simulink model "Latest_Greatest_vSandberg"  (R2022b)
settings: Solver=ode4  StartTime=0  StopTime=15  FixedStep=DeltaT  RelTol=1e-6  EnableMultiTasking=on
InitFcn:
  | %run('final_report_initexternal')
  | % Bifocal Relay Mirror Spacecraft (prior to payload installation) Dynamics Simulation          TA Sands
  | clear all;close all;clc;warning off all;
  | 
  | % Simulation run parameters
  | Rate=34.3; Rate=100;  DeltaT=1/Rate;
  | 
  | % Maneuver Parameters
  | roll=0;  pitch=0; yaw=30;   roll=roll*pi/180; pitch=pitch*pi/180; yaw=yaw*pi/180;
  | SlewStart=5; SlewTime=10; SACengage=0;
  | SlewStart=5; SlewTime=5;
  | t0=SlewTime;
  | tf=SlewTime+5;
  | %%
  | 
  | %Constants0
  | Re=6371.2e3;mu=398601.2e9;          %earth radius and universal gravitation constant
  | 
  | % tht=0.5*((sin(pi/SlewTime*(u(4)+2.5)))+1).*[u(1) u(2) u(3)]';
  | % w=(30/77.1239)*0.5*(pi/SlewTime)*((cos(pi/SlewTime*(u(4)+2.5)))+1).*[u(1) u(2) u(3)]'
  | % wdot=-(30/77.1239)*0.5*(pi/SlewTime)^(2)*((sin(pi/SlewTime*(u(4)+2.5)))).*[u(1) u(2) u(3)]'
  | 
  | %compare with differentiating in real time
  | 
  | % A0=[0 0 0];
  | % tht=A0+1/2*(1-cos(pi/SlewTime*(t-SlewStart)))*(A-A0);
  | % w=1/2*(pi/SlewTime)*sin(pi/SlewTime*(t-SlewStart))*(A-A0);
  | % wdot1=1/2*(pi/SlewTime)^2*cos(pi/SlewTime*(t-SlewStart))*(A-A0);
  | 
  | %Spacecraft orbit
  | h=0;                                     %orbit altitude
  | R=Re+h;                             %orbit radius from center of earth
  | we=0.000072921158553;   %earth's angular velocity rad/solar sec(Vallado)
  | wo=sqrt(mu/(Re+h)^3);        %orbit angular velocity
  | incln=36.6001*pi/180;          %Inclination assumed Monterey Latitude
  | epsilon=12*pi/180;  alphao=0;
  | uo=0; nuo=0;                        %Start S/C beneath subsolar point
  | betasun=60; gamma=1.5;
  | a=0.545491852; b=0.314939867;  c=0.704226952;   %Assumed spacecraft rectangular size
  | Area=[b*c a*c a*b];                 %projected area~m^2 in body x,y,z directions
  | density=4.39e-14;
  | kpre=-9.9639/24/3600/180*pi*0;      %nodal precession constant assumed zero here
  | wn=kpre*(Re/(Re+h))^3.5*cos(incln); %nodal precession (zero eccentricity)
  | V=wo*(Re+h);
  | rho=asin(Re/(h+Re));                %earth angular radius
  | Cd=2.5;     psun=4.5E-6;            %Drag coefficient and solar pressure constant~N/m^2
  | Kaero=-0.5*Cd*V^2;   Psolar=2*psun;  %constants for aero and solar torque calculation
  | dL=[0.002 0.002 0.008];             %predicted distance between cp and cg
  | Kme=2.3390e-005;
  | 
  | %Spacecraft Magnetic Properties (assumed)
  | mresid=[0 0 0.01];                  %Spacecraft residual magnetic moment
  | M=mresid;                           %Magnetic unit dipole vector
  | K=7.943e15;
  | 
  | %%
  | % Determining Principal Axes Frame
  | % ACTUAL Spacecraft Inertia conditions
  | Ix=16.67;   Iy=16.67;   Iz=16.67 ;
  | Ixy=0;  Iyz=0;  Ixz=0;
  | ... (+176 lines)
StopFcn:
  | toc
  | %run('final_report_stopexternal')
  | 
  | if flag==0; Hcmg=Hcmg;else;Hcmg=HcmgMP;end;
  | Hxcmg=[];Hycmg=[];Hzcmg=[];CondA=[]; CondA_MP=[];t=[]; SingPt=[];DetA=[];
  | for i=1:max(size(A));  t=[t i*DeltaT];  H=Hcmg(:,:,i); Hx=H(1,:);  Hy=H(2,:);  Hz=H(3,:);
  | detA=det(A(:,1:3,i));Hxcmg=[Hxcmg Hx];  Hycmg=[Hycmg Hy];  Hzcmg=[Hzcmg Hz];
  | CONDA=cond(A(:,:,i));
  | DetA=[DetA detA]; DetA=1./DetA;
  | CondA=[CondA CONDA];end;   %CondA=CondA./max(CondA); DetA=DetA./max(DetA);
  | Hmag=sqrt(Hxcmg.^2+Hycmg.^2+Hzcmg.^2);x=(max(t)-DeltaT);
  | 
  | InvCondA;
  | 
  | if flag==0; MaxInvCond=min(1./CondA(10*Rate+1:end));DELTA=delta;DELTAdot=deltadot;
  | else; MaxInvCond=min(1./CondA_MP(10*Rate+1:end));DELTA=delta_MP;DELTAdot=deltadot_MP;Hcmg=HcmgMP;end;
  | %
  | ERROR=(trajectory*180/pi-Euler);
  | 
  | figure(1); wdotTrajectory=[CMDTrajectory(:,1) CMDTrajectory(:,2) CMDTrajectory(:,3)];  wTrajectory=[CMDTrajectory(:,4) CMDTrajectory(:,5) CMDTrajectory(:,6)]; ThetaTrajectory=180/pi.*[trajectory(:,1) trajectory(:,2) trajectory(:,3)]; set(gca,'fontsize',32, 'fontname','Palatino Linotype');
  | subplot(3,1,1); plot(t,wdotTrajectory, 'linewidth',2); axis tight; grid; ylabel('\omega^d^o^t_C_M_D (deg)','fontsize',32); title('Desired Angle, Rate, Acceleration Trajectories','fontsize',32);   set(gca,'XTick',0:2:15);     set(gca,'XTickLabel',{' ',' ',' ',' ',' ',' ',' ',' ','15'}); set(gca,'fontsize',32, 'fontname','Palatino Linotype');
  | subplot(3,1,2); plot(t,wTrajectory,'linewidth',2); axis tight; grid; ylabel('\omega_C_M_D (deg)','fontsize',32);set(gca,'XTick',0:2:15);     set(gca,'XTickLabel',{' ',' ',' ',' ',' ',' ',' ',' ','15'}); set(gca,'fontsize',32, 'fontname','Palatino Linotype');
  | subplot(3,1,3); plot(t,ThetaTrajectory,'linewidth',2); axis tight; grid; ylabel('\theta_C_M_D (deg)','fontsize',32); xlabel('time (sec)','fontsize',32); set(gca,'fontsize',32, 'fontname','Palatino Linotype');
  | 
  | % figure(2);
  | % subplot(2,1,1);plot(t,Hmag,'LineWidth',3);   ylabel('|H_c_m_g|','Fontsize',16);grid;axis([0,x,0,3]); set(gca,'fontsize',16);set(gca,'XTickLabel',{' ',' ',' ',' ',' ',' ',' ',' ','15'});
  | % subplot(2,1,2);plot(t,InvCondA,'linewidth',3);grid;xlabel('t(sec)','fontsize',14,'fontname','times');ylabel('Cond[A]','fontsize',14,'fontname','times');axis([0,max(t),0,21.82]); set(gca,'fontsize',16);
  | %
  | % DELTA1=DELTA(1,:);DELTA2=DELTA(2,:);DELTA3=DELTA(3,:);DELTA4=DELTA(4,:);
  | % DELTAdot1=DELTAdot(1,:);DELTAdot2=DELTAdot(2,:);DELTAdot3=DELTAdot(3,:);DELTAdot4=DELTAdot(4,:);
  | %
  | % figure(3);subplot(4,1,1);plot(t,DELTA1,'LineWidth',3); title('Gimbal Angles','fontsize',16);ylabel('\theta_1(deg)','Fontsize',14);grid;axis tight; set(gca,'XTickLabel',{' ',' ',' ',' ',' ',' ',' ',' ','15'});set(gca,'fontsize',16);
  | % subplot(4,1,2);plot(t,DELTA2,'LineWidth',3); ylabel('\theta_2(deg)','Fontsize',16);grid;axis tight; set(gca,'XTickLabel',{' ',' ',' ',' ',' ',' ',' ',' ','15'});set(gca,'fontsize',16);
  | % subplot(4,1,3);plot(t,DELTA3,'LineWidth',3); ylabel('\theta_3(deg)','Fontsize',16);grid;axis tight; set(gca,'XTickLabel',{' ',' ',' ',' ',' ',' ',' ',' ','15'});set(gca,'fontsize',16);
  | % subplot(4,1,4);plot(t,InvCondA,'linewidth',3);grid;xlabel('t(sec)','fontsize',14,'fontname','times');ylabel('Cond[A]','fontsize',14,'fontname','times');axis([0,max(t),0,21.82]); set(gca,'fontsize',16);
  | %
  | % figure(4);subplot(4,1,1);plot(t,DELTAdot1,'LineWidth',3);  title('Gimbal Angle RATES','fontsize',16); ylabel('\theta_d_o_t_1(rad/s)','Fontsize',16);grid; axis([0,x,-pi*1.1,pi*1.1]);   set(gca,'XTickLabel',{' ',' ',' ',' ',' ',' ',' ',' ','15'});set(gca,'fontsize',16);
  | % subplot(4,1,2);plot(t,DELTAdot2,'LineWidth',3);   ylabel('\theta_d_o_t_2(rad/s)','Fontsize',16);grid;axis([0,x,-pi*1.1,pi*1.1]);   set(gca,'XTickLabel',{' ',' ',' ',' ',' ',' ',' ',' ','15'});   set(gca,'fontsize',16);
  | % subplot(4,1,3);plot(t,DELTAdot3,'LineWidth',3);   ylabel('\theta_d_o_t_3(rad/s)','Fontsize',16);grid;axis([0,x,-pi*1.1,pi*1.1]); set(gca,'XTickLabel',{' ',' ',' ',' ',' ',' ',' ',' ','15'});set(gca,'fontsize',16);
  | % subplot(4,1,4);plot(t,InvCondA,'linewidth',3);grid;xlabel('t(sec)','fontsize',14,'fontname','times');ylabel('Cond[A]','fontsize',14,'fontname','times');axis([0,max(t),0,21.82]); set(gca,'fontsize',16);
  | %
  | % figure(5);
  | % subplot(4,1,1);plot(t,Hxcmg,'linewidth',3);axis([0,x,-3.25,3.25]);grid;ylabel('h_x/|h|','fontsize',16);title('Normalized Momentum','fontsize',16);set(gca,'XTickLabel',{' ',' ',' ',' ',' ',' ',' ',' ','15'});set(gca,'fontsize',16);
  | % subplot(4,1,2);plot(t,Hycmg,'linewidth',3);axis([0,x,-3.25,3.25]);grid;ylabel('h_y/|h|','fontsize',16);set(gca,'XTickLabel',{' ',' ',' ',' ',' ',' ',' ',' ','15'});set(gca,'fontsize',16);
  | % subplot(4,1,3);plot(t,Hzcmg,'linewidth',3);axis([0,x,-3.25,3.25]);grid;ylabel('h_z/|h|','fontsize',16);  set(gca,'XTickLabel',{' ',' ',' ',' ',' ',' ',' ',' ','15'});set(gca,'fontsize',16);
  | % subplot(4,1,4);plot(t,InvCondA,'linewidth',3);grid;xlabel('t(sec)','fontsize',14,'fontname','times');ylabel('Cond[A]','fontsize',14,'fontname','times');axis([0,max(t),0,21.82]); set(gca,'fontsize',16);
  | %
  | figure(6); EulerX=Euler(:,1);EulerY=Euler(:,2);EulerZ=Euler(:,3);
  | subplot(4,1,1);plot(t,EulerX,'linewidth',3); axis([0,x,min(EulerX),max(EulerX)]);grid;ylabel('\phi(deg)','fontsize',32);title('True Euler Angles','fontsize',14);  set(gca,'XTickLabel',{' ',' ',' ',' ',' ',' ',' ',' ','15'});  set(gca,'fontsize',32, 'fontname','Palatino Linotype');
  | subplot(4,1,2);plot(t,EulerY,'linewidth',3);  axis([0,x,min(EulerY),max(EulerY)]); grid;ylabel('\theta(deg)','fontsize',32);  set(gca,'XTickLabel',{' ',' ',' ',' ',' ',' ',' ',' ','15'}); set(gca,'fontsize',32, 'fontname','Palatino Linotype');
  | subplot(4,1,3);plot(t,EulerZ,'linewidth',3);axis([0,x,min(EulerZ),max(EulerZ)]);grid;  ylabel('\psi(deg)','fontsize',32);  set(gca,'XTickLabel',{' ',' ',' ',' ',' ',' ',' ',' ','15'});  set(gca,'fontsize',32, 'fontname','Palatino Linotype');
  | subplot(4,1,4);plot(t,InvCondA,'linewidth',3);grid;xlabel('t(sec)','fontsize',32,'fontname','times');ylabel('Cond[A]','fontsize',14,'fontname','times');axis([0,max(t),0,21.82]); set(gca,'fontsize',32, 'fontname','Palatino Linotype');
  | 
  | EX=ERROR(:,1);  EY=ERROR(:,2);     EZ=ERROR(:,3);
  | MeanXerror=mean(EX); Xmean=num2str(MeanXerror); xmean=['\mu_\phi=', Xmean];
  | STDx=std(EX);Xsigma=num2str(STDx);SigmaX=['    \sigma_x=' Xsigma];  xlegend=[xmean, SigmaX];
  | MeanYerror=mean(EY); Ymean=num2str(MeanYerror); ymean=['\mu_\theta=', Ymean];
  | STDy=std(EY); Ysigma=num2str(STDy);SigmaY=['    \sigma_y=' Ysigma]; ylegend=[ymean, SigmaY];
  | MeanZerror=mean(EZ); Zmean=num2str(MeanZerror); zmean=['\mu_\psi=', Zmean];
  | STDz=std(EZ);Zsigma=num2str(STDz);SigmaZ=['    \sigma_z=' Zsigma]; zlegend=[zmean, SigmaZ];
  | ... (+113 lines)
undefined symbols (not defined in the file): magnitude, svd
libraries: vrlib x9, dspinverses x8, aerospace x5, matrix_library x4, simulink_need_slupdate x2, dspadpt3 x2
(part 2 of 4)

== system Latest_Greatest_vSandberg/Subsystem2/Subsystem1 ==
  note: DCM
  note: DCM
  note: Density needs to be fixed
  DCM : Inport
  r_body : Inport  Port=2
  Display : Display
  Gain : Gain
  Gravity Gradient1 : Subsystem
  Magnetic Torque : Subsystem
  On/Off : Gain  SaturateOnIntegerOverflow=on  OutDataTypeStr=Inherit: Same as input  ParamDataTypeStr=Inherit: Same as input
  "On/Off " : Gain  SaturateOnIntegerOverflow=on  OutDataTypeStr=Inherit: Same as input  ParamDataTypeStr=Inherit: Same as input
  On/off : Gain  SaturateOnIntegerOverflow=on  OutDataTypeStr=Inherit: Same as input  ParamDataTypeStr=Inherit: Same as input
  On/off1 : Gain  SaturateOnIntegerOverflow=on  OutDataTypeStr=Inherit: Same as input  ParamDataTypeStr=Inherit: Same as input
  Orbit parameters : Subsystem
  Scope : Scope
  TAero & Tsolar : Subsystem
  Magnetic Disturbance : Outport
  Aero & Solar Disturbances : Outport  Port=2
  Gravity Gradient Disturbance : Outport  Port=3
  Aero & Solar Disturbance Forces : Outport  Port=4
  Gravity Gradient Disturbance Force : Outport  Port=5
  wires:
  Gravity Gradient1/2(Fgg) -> Gain/1, Display/1, Scope/1
  On/off1/1 -> Aero & Solar Disturbance Forces/1
  r_body/1 -> Gravity Gradient1/2(r_body)
  Gravity Gradient1/1(Tgg) -> "On/Off "/1
  Gain/1 -> Gravity Gradient Disturbance Force/1
  TAero & Tsolar/2(Faero & Fsolar1) -> On/off1/1
  "On/Off "/1 -> Gravity Gradient Disturbance/1
  On/off/1 -> Aero & Solar Disturbances/1
  On/Off/1 -> Magnetic Disturbance/1
  Magnetic Torque/1(Sb) -> On/Off/1
  Orbit parameters/3(u) -> Magnetic Torque/4(u)
  Orbit parameters/2(incln) -> Magnetic Torque/3(inclination)
  Orbit parameters/1(alpha) -> Magnetic Torque/2(alpha)
  Orbit parameters/4(nu) -> TAero & Tsolar/1(nu)
  TAero & Tsolar/1(Taero & Tsolar) -> On/off/1
  DCM/1 -> Gravity Gradient1/1(DCM), TAero & Tsolar/2(DCM), Magnetic Torque/1(DCM)

== system Latest_Greatest_vSandberg/Subsystem3/Body Dynamics ==
  note: w
  note: N B
  note: Hs
  note: Hsdot
  note: [ ]
  note: Mx
      | My
      | Mz
  note: [ ]
  note: w
      | w
      | w
  note: x
      | y
      | z
  note: Spacecraft Dynamics
  T : Inport
  Cross Product : matrix_library/Cross Product
  H * Iinv : Gain  Gain=Iinv  Multiplication=Matrix(K*u)  SaturateOnIntegerOverflow=on  OutDataTypeStr=Inherit: Same as input  ParamDataTypeStr=Inherit: Same as input
  Hdot * Iinv : Gain  Gain=Iinv  Multiplication=Matrix(K*u)  SaturateOnIntegerOverflow=on  OutDataTypeStr=Inherit: Same as input  ParamDataTypeStr=Inherit: Same as input
  Integrator : Integrator
  Sum1 : Sum  Inputs=|++  InputSameDT=on  SaturateOnIntegerOverflow=on  OutDataTypeStr=Inherit: Same as first input
  To Workspace1 : ToWorkspace  VariableName=w  SampleTime=-1
  To Workspace2 : ToWorkspace  VariableName=wdot  SampleTime=-1
  h*[A] : Gain  Gain=1/h_wheel
  |H| : Fcn  Expr=sqrt(u[1]^2+u[2]^2+u[3]^2)
  |H| Display : Display
  |H| Scope : Scope
  NwB : Outport  VectorParamsAs1DForOutWhenUnconnected=off
  NwBdot : Outport  Port=2  VectorParamsAs1DForOutWhenUnconnected=off
  tag scope: hxw=global
  wires:
  Integrator/1 -> H * Iinv/1, Cross Product/1, |H|/1
  H * Iinv/1 -> Cross Product/2, NwB/1, To Workspace1/1
  Cross Product/1 -> [hxw], Sum1/2
  |H|/1 -> |H| Display/1, h*[A]/1
  Sum1/1 -> Integrator/1, Hdot * Iinv/1
  T/1 -> Sum1/1
  h*[A]/1 -> |H| Scope/1
  Hdot * Iinv/1 -> NwBdot/1, To Workspace2/1

== system Latest_Greatest_vSandberg/Subsystem3/Subsystem1 ==
  note: [ ]
  note: w
      | w
      | w
  note: x
      | y
      | z
  note: w
  note: N B
  note: w
  note: [ ]
  note: w
      | w
      | w
  note: 1
      | 2
      | 3
  note: w
  note: O B
  note: DCM
  note: N O
  note: [ ]
  note: f
      | q
      | y
  note: Spacecraft Kinematics
  wbn : Inport
  -wo : Gain  Gain=-wo  SaturateOnIntegerOverflow=on  OutDataTypeStr=Inherit: Same as input  ParamDataTypeStr=Inherit: Same as input
  -wo1 : Gain  Gain=0  SaturateOnIntegerOverflow=on  OutDataTypeStr=Inherit: Same as input  ParamDataTypeStr=Inherit: Same as input
  Euler Angle : Subsystem
  Quaternion Kinematics : Subsystem
  Select ci2 : Subsystem
  Sum : Sum  Inputs=-+|  InputSameDT=on  SaturateOnIntegerOverflow=on  OutDataTypeStr=Inherit: Same as first input
  To Workspace : ToWorkspace  VariableName=Euler  SampleTime=-1
  rad2deg : Gain  Gain=180/pi  SaturateOnIntegerOverflow=on  OutDataTypeStr=Inherit: Same as input  ParamDataTypeStr=Inherit: Same as input
  DCM : Outport  VectorParamsAs1DForOutWhenUnconnected=off
  Euler(deg) : Outport  Port=2  VectorParamsAs1DForOutWhenUnconnected=off
  Euler(rad) : Outport  Port=3  VectorParamsAs1DForOutWhenUnconnected=off
  wires:
  Sum/1 -> Quaternion Kinematics/1(OwB)
  -wo/1 -> -wo1/1
  Select ci2/1(U(E)) -> -wo/1
  Quaternion Kinematics/1(DCM) -> Euler Angle/1(DCM1), Select ci2/1(U), DCM/1
  -wo1/1 -> Sum/1
  wbn/1 -> Sum/2
  Euler Angle/1(Euler Angles1) -> rad2deg/1, Euler(rad)/1
  rad2deg/1 -> Euler(deg)/1, To Workspace/1

== system Latest_Greatest_vSandberg/Subsystem5/OBSERVERS (MASK THIS SUBSYSTEM AS CLASS DEMO)1 ==
  Full State Feedback : Inport
  Demux : Demux  Outputs=2
  Subsystem : Subsystem
      mask Display: disp('Luenberger & PID Observers')
  Terminator : Terminator
  Estimated full state feedback (Euler-rad) : Outport  VectorParamsAs1DForOutWhenUnconnected=off
  wires:
  Demux/1 -> Subsystem/1(Euler Angle (rad))
  Demux/2 -> Terminator/1
  Subsystem/1(Estimated Full State Feedback) -> Estimated full state feedback (Euler-rad)/1
  Full State Feedback/1 -> Demux/1

== system Latest_Greatest_vSandberg/Subsystem5/Subsystem2 ==
  note: Noisy Sensor
  Full State Feedback : Inport
  Random Number : RandomNumber  Variance=NoiseVariance  SampleTime=0
  Sum1 : Sum  Inputs=|++
  Noisy State Feedback : Outport  VectorParamsAs1DForOutWhenUnconnected=off
  wires:
  Random Number/1 -> Sum1/2
  Sum1/1 -> Noisy State Feedback/1
  Full State Feedback/1 -> Sum1/1

== system Latest_Greatest_vSandberg/Subsystem5/Subsystem4 ==
  Full State Feedback : Inport
  Demux : Demux  Outputs=2
  Filter Error (deg) : Scope
      settings: StopFcn=|
      | %Simulink figure properties
      | shh=get(0,'ShowHiddenHandles');
      | set(0,'ShowHiddenHandles','On')
      | set(gcf,'menubar','figure')
      | set(gcf,'CloseRequestFcn','closereq')
      | set(gcf,'DefaultLineClipping','Off')
      | set(0,'ShowHiddenHandles',shh)
  Filtered Euler Angles (deg) : Scope
      settings: StopFcn=|
      | %Simulink figure properties
      | shh=get(0,'ShowHiddenHandles');
      | set(0,'ShowHiddenHandles','On')
      | set(gcf,'menubar','figure')
      | set(gcf,'CloseRequestFcn','closereq')
      | set(gcf,'DefaultLineClipping','Off')
      | set(0,'ShowHiddenHandles',shh)
  Kalman Filter : dspadpt3/Kalman Filter  num_targets=1  sourceEnable=Always  isReset=on  X=zeros([3, 1])  P=10*eye(3)  A=eye(3)  sourceMeasure=Specify via Dialog  H=eye(3)  Q=0.05*eye(3)  R=eye(3)  isOutputEstMeasure=off  isOutputEstState=on  isOutputEstError=off  isOutputPrdMeasure=off  isOutputPrdState=off  isOutputPrdError=off
  Kalman Filter1 : dspadpt3/Kalman Filter  num_targets=1  sourceEnable=Always  isReset=on  X=zeros([3, 1])  P=10*eye(3)  A=eye(3)  sourceMeasure=Specify via Dialog  H=eye(3)  Q=0.05*eye(3)  R=eye(3)  isOutputEstMeasure=off  isOutputEstState=on  isOutputEstError=off  isOutputPrdMeasure=off  isOutputPrdState=off  isOutputPrdError=off
  Mux : Mux  Inputs=2
  Reshape : Reshape
  Sum3 : Sum  Inputs=|+-
  To Workspace : ToWorkspace  VariableName=FilteredEuler  SampleTime=-1
  To Workspace2 : ToWorkspace  VariableName=KalmanEstimationError  SampleTime=-1
  degrees-to-radians2 : Gain  Gain=180/pi
  Out1 : Outport  VectorParamsAs1DForOutWhenUnconnected=off
  wires:
  [ActualEuler] -> Sum3/1
  Reshape/1 -> Sum3/2
  Sum3/1 -> Filter Error (deg)/1, To Workspace2/1
  degrees-to-radians2/1 -> Reshape/1, To Workspace/1, Filtered Euler Angles (deg)/1
  Kalman Filter/1 -> degrees-to-radians2/1, Mux/1
  Demux/2 -> Kalman Filter1/1
  Full State Feedback/1 -> Demux/1
  Demux/1 -> Kalman Filter/1
  Mux/1 -> Out1/1
  Kalman Filter1/1 -> Mux/2

== system Latest_Greatest_vSandberg/Subsystem5/Subsystem5 ==
  note: See Bong Wie
      | Generalized Second Order Filters
      | 2nd Edition pg 137
  u : Inport
  Demux : Demux  Outputs=6
  Mux : Mux  Inputs=6
  Transfer Fcn{,1..5} (6 alike) : TransferFcn  Numerator="[1/wz^2   2*dampZ/wz  1]"  Denominator="[1/wp^2   2*dampP/wp  1]"
  u(filtered) : Outport  VectorParamsAs1DForOutWhenUnconnected=off
  wires:
  Mux/1 -> u(filtered)/1
  u/1 -> Demux/1
  Transfer Fcn/1 -> Mux/1
  Transfer Fcn1/1 -> Mux/2
  Transfer Fcn2/1 -> Mux/3
  Transfer Fcn3/1 -> Mux/4
  Transfer Fcn4/1 -> Mux/5
  Transfer Fcn5/1 -> Mux/6
  Demux/1 -> Transfer Fcn/1
  Demux/2 -> Transfer Fcn1/1
  Demux/3 -> Transfer Fcn2/1
  Demux/4 -> Transfer Fcn3/1
  Demux/5 -> Transfer Fcn4/1
  Demux/6 -> Transfer Fcn5/1

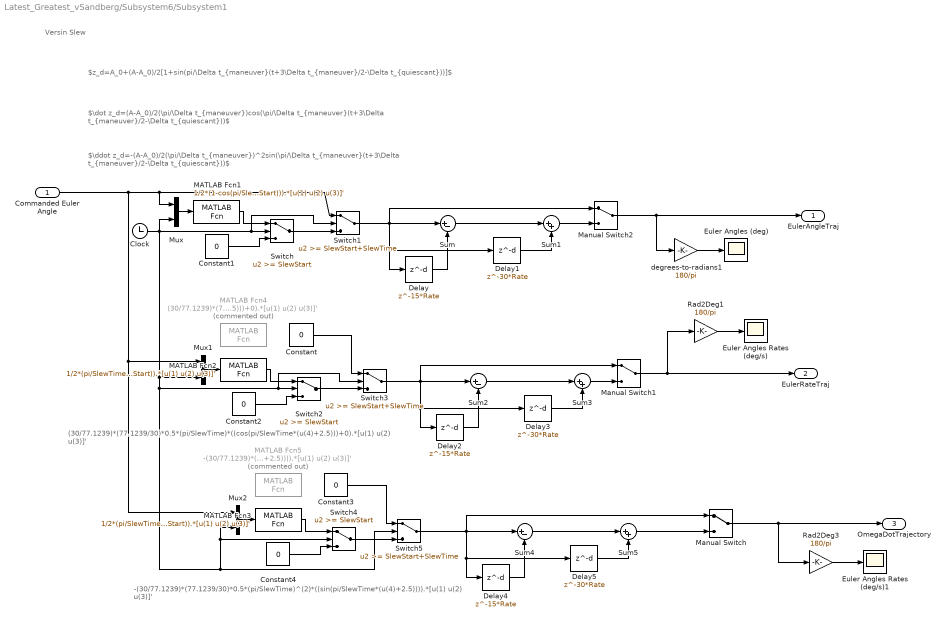
== system Latest_Greatest_vSandberg/Subsystem6/Subsystem1 ==
  note: (30/77.1239)*(77.1239/30)*0.5*(pi/SlewTime)*((cos(pi/SlewTime*(u(4)+2.5)))+0).*[u(1) u(2) u(3)]'
  note: -(30/77.1239)*(77.1239/30)*0.5*(pi/SlewTime)^(2)*((sin(pi/SlewTime*(u(4)+2.5)))).*[u(1) u(2) u(3)]'
  note: Versin Slew
  note: $z_d=A_0+(A-A_0)/2[1+sin(pi/\Delta t_{maneuver}(t+3\Delta t_{maneuver}/2-\Delta t_{quiescant}))]$
  note: $\dot z_d=(A-A_0)/2(\pi/\Delta t_{maneuver})cos(\pi/\Delta t_{maneuver}(t+3\Delta t_{maneuver}/2-\Delta t_{quiescant}))$
  note: $\ddot z_d=-(A-A_0)/2(\pi/\Delta t_{maneuver})^2sin(\pi/\Delta t_{maneuver}(t+3\Delta t_{maneuver}/2-\Delta t_{quiescant}))$
  Commanded Euler Angle : Inport
  Clock : Clock
  Constant{,1..4} (5 alike) : Constant  Value=0
  Delay : Delay  DelayLength=15*Rate
  Delay1 : Delay  DelayLength=30*Rate
  Delay2 : Delay  DelayLength=15*Rate
  Delay3 : Delay  DelayLength=30*Rate
  Delay4 : Delay  DelayLength=15*Rate
  Delay5 : Delay  DelayLength=30*Rate
  Euler Angles (deg) : Scope
      settings: StopFcn=|
      | %Simulink figure properties
      | shh=get(0,'ShowHiddenHandles');
      | set(0,'ShowHiddenHandles','On')
      | set(gcf,'menubar','figure')
      | set(gcf,'CloseRequestFcn','closereq')
      | set(gcf,'DefaultLineClipping','Off')
      | set(0,'ShowHiddenHandles',shh)
  Euler Angles Rates (deg/s) : Scope
      settings: StopFcn=|
      | %Simulink figure properties
      | shh=get(0,'ShowHiddenHandles');
      | set(0,'ShowHiddenHandles','On')
      | set(gcf,'menubar','figure')
      | set(gcf,'CloseRequestFcn','closereq')
      | set(gcf,'DefaultLineClipping','Off')
      | set(0,'ShowHiddenHandles',shh)
  Euler Angles Rates (deg/s)1 : Scope
      settings: StopFcn=|
      | %Simulink figure properties
      | shh=get(0,'ShowHiddenHandles');
      | set(0,'ShowHiddenHandles','On')
      | set(gcf,'menubar','figure')
      | set(gcf,'CloseRequestFcn','closereq')
      | set(gcf,'DefaultLineClipping','Off')
      | set(0,'ShowHiddenHandles',shh)
  MATLAB Fcn1 : MATLABFcn  MATLABFcn=1/2*(1-cos(pi/SlewTime*(u(4)-SlewStart))).*[u(1) u(2) u(3)]'
  MATLAB Fcn2 : MATLABFcn  MATLABFcn=1/2*(pi/SlewTime)*sin(pi/SlewTime*(u(4)-SlewStart)).*[u(1) u(2) u(3)]'
  MATLAB Fcn3 : MATLABFcn  MATLABFcn=1/2*(pi/SlewTime)^2*cos(pi/SlewTime*(u(4)-SlewStart)).*[u(1) u(2) u(3)]'
  MATLAB Fcn4 : MATLABFcn  Commented=on  MATLABFcn=(30/77.1239)*(77.1239/30)*0.5*(pi/SlewTime)*((cos(pi/SlewTime*(u(4)+2.5)))+0).*[u(1) u(2) u(3)]'
  MATLAB Fcn5 : MATLABFcn  Commented=on  MATLABFcn=-(30/77.1239)*(77.1239/30)*0.5*(pi/SlewTime)^(2)*((sin(pi/SlewTime*(u(4)+2.5)))).*[u(1) u(2) u(3)]'
  Manual Switch : ManualSwitch
  Manual Switch1 : ManualSwitch
  Manual Switch2 : ManualSwitch
  Mux : Mux  Inputs=2
  Mux1 : Mux  Inputs=2
  Mux2 : Mux  Inputs=2
  Rad2Deg1 : Gain  Gain=180/pi
  Rad2Deg3 : Gain  Gain=180/pi
  Sum : Sum  Inputs=|+-
  Sum1 : Sum  Inputs=|++
  Sum2 : Sum  Inputs=|+-
  Sum3 : Sum  Inputs=|++
  Sum4 : Sum  Inputs=|+-
  Sum5 : Sum  Inputs=|++
  Switch : Switch  Threshold=SlewStart  SaturateOnIntegerOverflow=off  InputSameDT=off
  Switch1 : Switch  Threshold=SlewStart+SlewTime  SaturateOnIntegerOverflow=off  InputSameDT=off
  Switch2 : Switch  Threshold=SlewStart  SaturateOnIntegerOverflow=off  InputSameDT=off
  Switch3 : Switch  Threshold=SlewStart+SlewTime  SaturateOnIntegerOverflow=off  InputSameDT=off
  Switch4 : Switch  Threshold=SlewStart  SaturateOnIntegerOverflow=off  InputSameDT=off
  Switch5 : Switch  Threshold=SlewStart+SlewTime  SaturateOnIntegerOverflow=off  InputSameDT=off
  degrees-to-radians1 : Gain  Gain=180/pi
  EulerAngleTraj : Outport  VectorParamsAs1DForOutWhenUnconnected=off
  EulerRateTraj : Outport  Port=2  VectorParamsAs1DForOutWhenUnconnected=off
  OmegaDotTrajectory : Outport  Port=3  VectorParamsAs1DForOutWhenUnconnected=off
  wires:
  Mux2/1 -> MATLAB Fcn3/1
  MATLAB Fcn3/1 -> Switch4/1
  Constant4/1 -> Switch4/3
  Switch4/1 -> Switch5/3
  Constant3/1 -> Switch5/1
  Constant/1 -> Switch3/1
  Switch2/1 -> Switch3/3
  Constant2/1 -> Switch2/3
  MATLAB Fcn2/1 -> Switch2/1
  Mux1/1 -> MATLAB Fcn2/1
  Rad2Deg1/1 -> Euler Angles Rates (deg/s)/1
  degrees-to-radians1/1 -> Euler Angles (deg)/1
  Mux/1 -> MATLAB Fcn1/1
  Commanded Euler Angle/1 -> Mux2/1, Mux1/1, Switch1/1, Mux/1
  MATLAB Fcn1/1 -> Switch/1
  Clock/1 -> Switch5/2, Switch4/2, Mux2/2, Switch2/2, Switch3/2, Mux1/2, Mux/2, Switch1/2, Switch/2
  Constant1/1 -> Switch/3
  Switch/1 -> Switch1/3
  Switch1/1 -> Manual Switch2/1, Sum/1, Delay/1, Delay1/1
  Rad2Deg3/1 -> Euler Angles Rates (deg/s)1/1
  Delay/1 -> Sum/2
  Sum/1 -> Sum1/1
  Delay1/1 -> Sum1/2
  Delay2/1 -> Sum2/2
  Delay3/1 -> Sum3/2
  Switch3/1 -> Manual Switch1/1, Sum2/1, Delay2/1, Delay3/1
  Sum2/1 -> Sum3/1
  Delay4/1 -> Sum4/2
  Delay5/1 -> Sum5/2
  Switch5/1 -> Sum4/1, Manual Switch/1, Delay4/1, Delay5/1
  Sum4/1 -> Sum5/1
  Manual Switch/1 -> Rad2Deg3/1, OmegaDotTrajectory/1
  Sum5/1 -> Manual Switch/2
  Manual Switch1/1 -> EulerRateTraj/1, Rad2Deg1/1
  Sum3/1 -> Manual Switch1/2
  Sum1/1 -> Manual Switch2/2
  Manual Switch2/1 -> EulerAngleTraj/1, degrees-to-radians1/1

== system Latest_Greatest_vSandberg/Subsystem6/Subsystem2 ==
  In1 : Inport
  Demux : Demux  Outputs=3
  To Workspace1 : ToWorkspace  VariableName=roll  SampleTime=-1
  To Workspace2 : ToWorkspace  VariableName=pitch  SampleTime=-1
  To Workspace3 : ToWorkspace  VariableName=yaw  SampleTime=-1
  wires:
  In1/1 -> Demux/1
  Demux/1 -> To Workspace1/1
  Demux/2 -> To Workspace2/1
  Demux/3 -> To Workspace3/1

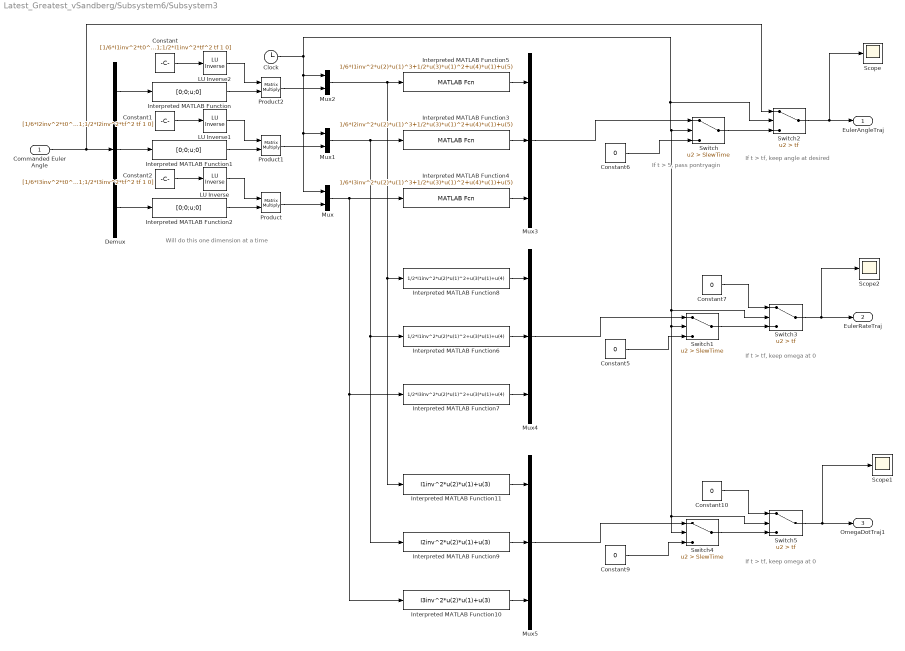
== system Latest_Greatest_vSandberg/Subsystem6/Subsystem3 ==
  note: If t > tf, keep omega at 0
  note: Will do this one dimension at a time
  note: If t > 5, pass pontryagin
  note: If t > tf, keep angle at desired
  note: If t > tf, keep omega at 0
  Commanded Euler Angle : Inport
  " LU Inverse" : dspinverses/ LU Inverse
  " LU Inverse1" : dspinverses/ LU Inverse
  " LU Inverse2" : dspinverses/ LU Inverse
  Clock : Clock
  Constant : Constant  Value=[1/6*I1inv^2*t0^3 1/2*t0^2 t0 1;1/2*I1inv^2*t0^2 t0 1 0;1/6*I1inv^2*tf^3 1/2*tf^2 tf 1;1/2*I1inv^2*tf^2 tf 1 0]
      mask Display: disp('[T1]')
  Constant1 : Constant  Value=[1/6*I2inv^2*t0^3 1/2*t0^2 t0 1;1/2*I2inv^2*t0^2 t0 1 0;1/6*I2inv^2*tf^3 1/2*tf^2 tf 1;1/2*I2inv^2*tf^2 tf 1 0]
      mask Display: disp('[T2]')
  Constant{5..7,9..10} (5 alike) : Constant  Value=0
  Constant2 : Constant  Value=[1/6*I3inv^2*t0^3 1/2*t0^2 t0 1;1/2*I3inv^2*t0^2 t0 1 0;1/6*I3inv^2*tf^3 1/2*tf^2 tf 1;1/2*I3inv^2*tf^2 tf 1 0]
      mask Display: disp('[T3]')
  Demux : Demux  Outputs=3
  Interpreted MATLAB Function : MATLABFcn  MATLABFcn=[0;0;u;0]
      mask Display: disp('[b]=[theta0;w0;thetaf;wf]')
  Interpreted MATLAB Function1 : MATLABFcn  MATLABFcn=[0;0;u;0]
      mask Display: disp('[b]=[theta0;w0;thetaf;wf]')
  Interpreted MATLAB Function10 : MATLABFcn  MATLABFcn=I3inv^2*u(2)*u(1)+u(3)
      mask Display: disp('wdot3=a/I3*t+b')
  Interpreted MATLAB Function11 : MATLABFcn  MATLABFcn=I1inv^2*u(2)*u(1)+u(3)
      mask Display: disp('wdot1=a/I1*t+b')
  Interpreted MATLAB Function2 : MATLABFcn  MATLABFcn=[0;0;u;0]
      mask Display: disp('[b]=[theta0;w0;thetaf;wf]')
  Interpreted MATLAB Function3 : MATLABFcn  MATLABFcn=1/6*I2inv^2*u(2)*u(1)^3+1/2*u(3)*u(1)^2+u(4)*u(1)+u(5)
      mask Display: disp('psi=1/6*1/I2*at^3+1/2bt^2+ct+d')
  Interpreted MATLAB Function4 : MATLABFcn  MATLABFcn=1/6*I3inv^2*u(2)*u(1)^3+1/2*u(3)*u(1)^2+u(4)*u(1)+u(5)
      mask Display: disp('psi=1/6*1/I3*at^3+1/2bt^2+ct+d')
  Interpreted MATLAB Function5 : MATLABFcn  MATLABFcn=1/6*I1inv^2*u(2)*u(1)^3+1/2*u(3)*u(1)^2+u(4)*u(1)+u(5)
      mask Display: disp('tht=1/6*1/I1*at^3+1/2bt^2+ct+d')
  Interpreted MATLAB Function6 : MATLABFcn  MATLABFcn=1/2*I1inv^2*u(2)*u(1)^2+u(3)*u(1)+u(4)
      mask Display: disp('w2=1/2*1/I2*at^2+bt+c')
  Interpreted MATLAB Function7 : MATLABFcn  MATLABFcn=1/2*I3inv^2*u(2)*u(1)^2+u(3)*u(1)+u(4)
      mask Display: disp('w3=1/2*1/I3*at^2+bt+c')
  Interpreted MATLAB Function8 : MATLABFcn  MATLABFcn=1/2*I1inv^2*u(2)*u(1)^2+u(3)*u(1)+u(4)
      mask Display: disp('w1=1/2*1/I1*at^2+bt+c')
  Interpreted MATLAB Function9 : MATLABFcn  MATLABFcn=I2inv^2*u(2)*u(1)+u(3)
      mask Display: disp('wdot2=a/I12*t+b')
  Mux : Mux  Inputs=2
  Mux1 : Mux  Inputs=2
  Mux2 : Mux  Inputs=2
  Mux3 : Mux  Inputs=3
  Mux4 : Mux  Inputs=3
  Mux5 : Mux  Inputs=3
  Product : Product  Multiplication=Matrix(*)
  Product1 : Product  Multiplication=Matrix(*)
  Product2 : Product  Multiplication=Matrix(*)
  Scope : Scope
  Scope1 : Scope
  Scope2 : Scope
  Switch : Switch  Criteria=u2 > Threshold  Threshold=SlewTime  SaturateOnIntegerOverflow=off  InputSameDT=off
  Switch1 : Switch  Criteria=u2 > Threshold  Threshold=SlewTime  SaturateOnIntegerOverflow=off  InputSameDT=off
  Switch2 : Switch  Criteria=u2 > Threshold  Threshold=tf  SaturateOnIntegerOverflow=off  InputSameDT=off
  Switch3 : Switch  Criteria=u2 > Threshold  Threshold=tf  SaturateOnIntegerOverflow=off  InputSameDT=off
  Switch4 : Switch  Criteria=u2 > Threshold  Threshold=SlewTime  SaturateOnIntegerOverflow=off  InputSameDT=off
  Switch5 : Switch  Criteria=u2 > Threshold  Threshold=tf  SaturateOnIntegerOverflow=off  InputSameDT=off
  EulerAngleTraj : Outport  VectorParamsAs1DForOutWhenUnconnected=off
  EulerRateTraj : Outport  Port=2  VectorParamsAs1DForOutWhenUnconnected=off
  OmegaDotTraj1 : Outport  Port=3  VectorParamsAs1DForOutWhenUnconnected=off
  wires:
  Interpreted MATLAB Function11/1 -> Mux5/1
  Interpreted MATLAB Function9/1 -> Mux5/2
  Mux2/1 -> Interpreted MATLAB Function5/1, Interpreted MATLAB Function11/1, Interpreted MATLAB Function8/1
  Mux1/1 -> Interpreted MATLAB Function9/1, Interpreted MATLAB Function6/1, Interpreted MATLAB Function3/1
  Interpreted MATLAB Function10/1 -> Mux5/3
  Switch4/1 -> Switch5/3
  Constant9/1 -> Switch4/3
  Clock/1 -> Mux/1, Mux1/1, Mux2/1, Switch/2, Switch1/2, Switch4/2, Switch5/2, Switch3/2, Switch2/2
  Mux/1 -> Interpreted MATLAB Function10/1, Interpreted MATLAB Function7/1, Interpreted MATLAB Function4/1
  Constant10/1 -> Switch5/1
  Switch5/1 -> OmegaDotTraj1/1, Scope1/1
  Mux5/1 -> Switch4/1
  Switch3/1 -> EulerRateTraj/1, Scope2/1
  Switch2/1 -> EulerAngleTraj/1, Scope/1
  Constant7/1 -> Switch3/1
  Switch/1 -> Switch2/3
  Switch1/1 -> Switch3/3
  Constant6/1 -> Switch/3
  Constant5/1 -> Switch1/3
  Mux4/1 -> Switch1/1
  Mux3/1 -> Switch/1
  Interpreted MATLAB Function8/1 -> Mux4/1
  Interpreted MATLAB Function7/1 -> Mux4/3
  Interpreted MATLAB Function6/1 -> Mux4/2
  Interpreted MATLAB Function3/1 -> Mux3/2
  Interpreted MATLAB Function4/1 -> Mux3/3
  Interpreted MATLAB Function5/1 -> Mux3/1
  Product2/1 -> Mux2/2
  Product1/1 -> Mux1/2
  Product/1 -> Mux/2
  Interpreted MATLAB Function1/1 -> Product1/2
  " LU Inverse1"/1 -> Product1/1
  " LU Inverse2"/1 -> Product2/1
  Interpreted MATLAB Function/1 -> Product2/2
  Interpreted MATLAB Function2/1 -> Product/2
  " LU Inverse"/1 -> Product/1
  Constant2/1 -> " LU Inverse"/1
  Constant1/1 -> " LU Inverse1"/1
  Constant/1 -> " LU Inverse2"/1
  Demux/3 -> Interpreted MATLAB Function2/1
  Demux/2 -> Interpreted MATLAB Function1/1
  Demux/1 -> Interpreted MATLAB Function/1
  Commanded Euler Angle/1 -> Demux/1, Switch2/1

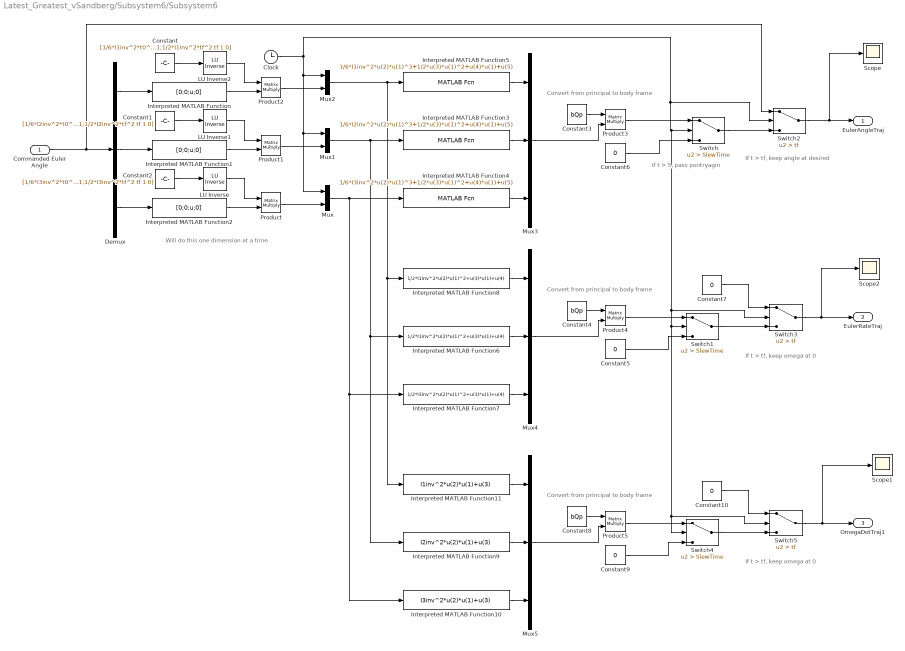
== system Latest_Greatest_vSandberg/Subsystem6/Subsystem6 ==
  note: If t > tf, keep omega at 0
  note: If t > tf, keep angle at desired
  note: If t > 5, pass pontryagin
  note: Convert from principal to body frame
  note: Will do this one dimension at a time
  note: Convert from principal to body frame
  note: Convert from principal to body frame
  note: If t > tf, keep omega at 0
  Commanded Euler Angle : Inport
  " LU Inverse" : dspinverses/ LU Inverse
  " LU Inverse1" : dspinverses/ LU Inverse
  " LU Inverse2" : dspinverses/ LU Inverse
  Clock : Clock
  Constant : Constant  Value=[1/6*I1inv^2*t0^3 1/2*t0^2 t0 1;1/2*I1inv^2*t0^2 t0 1 0;1/6*I1inv^2*tf^3 1/2*tf^2 tf 1;1/2*I1inv^2*tf^2 tf 1 0]
      mask Display: disp('[T1]')
  Constant1 : Constant  Value=[1/6*I2inv^2*t0^3 1/2*t0^2 t0 1;1/2*I2inv^2*t0^2 t0 1 0;1/6*I2inv^2*tf^3 1/2*tf^2 tf 1;1/2*I2inv^2*tf^2 tf 1 0]
      mask Display: disp('[T2]')
  Constant{5..7,9..10} (5 alike) : Constant  Value=0
  Constant2 : Constant  Value=[1/6*I3inv^2*t0^3 1/2*t0^2 t0 1;1/2*I3inv^2*t0^2 t0 1 0;1/6*I3inv^2*tf^3 1/2*tf^2 tf 1;1/2*I3inv^2*tf^2 tf 1 0]
      mask Display: disp('[T3]')
  Constant3 : Constant  Value=bQp
  Constant4 : Constant  Value=bQp
  Constant8 : Constant  Value=bQp
  Demux : Demux  Outputs=3
  Interpreted MATLAB Function : MATLABFcn  MATLABFcn=[0;0;u;0]
      mask Display: disp('[b]=[theta0;w0;thetaf;wf]')
  Interpreted MATLAB Function1 : MATLABFcn  MATLABFcn=[0;0;u;0]
      mask Display: disp('[b]=[theta0;w0;thetaf;wf]')
  Interpreted MATLAB Function10 : MATLABFcn  MATLABFcn=I3inv^2*u(2)*u(1)+u(3)
      mask Display: disp('wdot3=a/I3*t+b')
  Interpreted MATLAB Function11 : MATLABFcn  MATLABFcn=I1inv^2*u(2)*u(1)+u(3)
      mask Display: disp('wdot1=a/I1*t+b')
  Interpreted MATLAB Function2 : MATLABFcn  MATLABFcn=[0;0;u;0]
      mask Display: disp('[b]=[theta0;w0;thetaf;wf]')
  Interpreted MATLAB Function3 : MATLABFcn  MATLABFcn=1/6*I2inv^2*u(2)*u(1)^3+1/2*u(3)*u(1)^2+u(4)*u(1)+u(5)
      mask Display: disp('psi=1/6*1/I2*at^3+1/2bt^2+ct+d')
  Interpreted MATLAB Function4 : MATLABFcn  MATLABFcn=1/6*I3inv^2*u(2)*u(1)^3+1/2*u(3)*u(1)^2+u(4)*u(1)+u(5)
      mask Display: disp('psi=1/6*1/I3*at^3+1/2bt^2+ct+d')
  Interpreted MATLAB Function5 : MATLABFcn  MATLABFcn=1/6*I1inv^2*u(2)*u(1)^3+1/2*u(3)*u(1)^2+u(4)*u(1)+u(5)
      mask Display: disp('tht=1/6*1/I1*at^3+1/2bt^2+ct+d')
  Interpreted MATLAB Function6 : MATLABFcn  MATLABFcn=1/2*I1inv^2*u(2)*u(1)^2+u(3)*u(1)+u(4)
      mask Display: disp('w2=1/2*1/I2*at^2+bt+c')
  Interpreted MATLAB Function7 : MATLABFcn  MATLABFcn=1/2*I3inv^2*u(2)*u(1)^2+u(3)*u(1)+u(4)
      mask Display: disp('w3=1/2*1/I3*at^2+bt+c')
  Interpreted MATLAB Function8 : MATLABFcn  MATLABFcn=1/2*I1inv^2*u(2)*u(1)^2+u(3)*u(1)+u(4)
      mask Display: disp('w1=1/2*1/I1*at^2+bt+c')
  Interpreted MATLAB Function9 : MATLABFcn  MATLABFcn=I2inv^2*u(2)*u(1)+u(3)
      mask Display: disp('wdot2=a/I12*t+b')
  Mux : Mux  Inputs=2
  Mux1 : Mux  Inputs=2
  Mux2 : Mux  Inputs=2
  Mux3 : Mux  Inputs=3
  Mux4 : Mux  Inputs=3
  Mux5 : Mux  Inputs=3
  Product{,1..5} (6 alike) : Product  Multiplication=Matrix(*)
  Scope : Scope
  Scope1 : Scope
  Scope2 : Scope
  Switch : Switch  Criteria=u2 > Threshold  Threshold=SlewTime  SaturateOnIntegerOverflow=off  InputSameDT=off
  Switch1 : Switch  Criteria=u2 > Threshold  Threshold=SlewTime  SaturateOnIntegerOverflow=off  InputSameDT=off
  Switch2 : Switch  Criteria=u2 > Threshold  Threshold=tf  SaturateOnIntegerOverflow=off  InputSameDT=off
  Switch3 : Switch  Criteria=u2 > Threshold  Threshold=tf  SaturateOnIntegerOverflow=off  InputSameDT=off
  Switch4 : Switch  Criteria=u2 > Threshold  Threshold=SlewTime  SaturateOnIntegerOverflow=off  InputSameDT=off
  Switch5 : Switch  Criteria=u2 > Threshold  Threshold=tf  SaturateOnIntegerOverflow=off  InputSameDT=off
  EulerAngleTraj : Outport  VectorParamsAs1DForOutWhenUnconnected=off
  EulerRateTraj : Outport  Port=2  VectorParamsAs1DForOutWhenUnconnected=off
  OmegaDotTraj1 : Outport  Port=3  VectorParamsAs1DForOutWhenUnconnected=off
  wires:
  Commanded Euler Angle/1 -> Switch2/1, Demux/1
  Demux/1 -> Interpreted MATLAB Function/1
  Demux/2 -> Interpreted MATLAB Function1/1
  Demux/3 -> Interpreted MATLAB Function2/1
  Constant/1 -> " LU Inverse2"/1
  Constant1/1 -> " LU Inverse1"/1
  Constant2/1 -> " LU Inverse"/1
  " LU Inverse"/1 -> Product/1
  Interpreted MATLAB Function2/1 -> Product/2
  Interpreted MATLAB Function/1 -> Product2/2
  " LU Inverse2"/1 -> Product2/1
  " LU Inverse1"/1 -> Product1/1
  Interpreted MATLAB Function1/1 -> Product1/2
  Product/1 -> Mux/2
  Product1/1 -> Mux1/2
  Product2/1 -> Mux2/2
  Interpreted MATLAB Function5/1 -> Mux3/1
  Mux3/1 -> Product3/2
  Interpreted MATLAB Function4/1 -> Mux3/3
  Interpreted MATLAB Function3/1 -> Mux3/2
  Constant3/1 -> Product3/1
  Constant4/1 -> Product4/1
  Interpreted MATLAB Function6/1 -> Mux4/2
  Interpreted MATLAB Function7/1 -> Mux4/3
  Mux4/1 -> Product4/2
  Interpreted MATLAB Function8/1 -> Mux4/1
  Product3/1 -> Switch/1
  Product4/1 -> Switch1/1
  Constant5/1 -> Switch1/3
  Constant6/1 -> Switch/3
  Switch1/1 -> Switch3/3
  Switch/1 -> Switch2/3
  Constant7/1 -> Switch3/1
  Switch2/1 -> Scope/1, EulerAngleTraj/1
  Switch3/1 -> Scope2/1, EulerRateTraj/1
  Product5/1 -> Switch4/1
  Switch5/1 -> Scope1/1, OmegaDotTraj1/1
  Constant10/1 -> Switch5/1
  Mux5/1 -> Product5/2
  Mux/1 -> Interpreted MATLAB Function4/1, Interpreted MATLAB Function7/1, Interpreted MATLAB Function10/1
  Clock/1 -> Switch2/2, Switch3/2, Switch5/2, Switch4/2, Switch1/2, Switch/2, Mux2/1, Mux1/1, Mux/1
  Constant9/1 -> Switch4/3
  Switch4/1 -> Switch5/3
  Interpreted MATLAB Function10/1 -> Mux5/3
  Mux1/1 -> Interpreted MATLAB Function3/1, Interpreted MATLAB Function6/1, Interpreted MATLAB Function9/1
  Constant8/1 -> Product5/1
  Mux2/1 -> Interpreted MATLAB Function8/1, Interpreted MATLAB Function11/1, Interpreted MATLAB Function5/1
  Interpreted MATLAB Function9/1 -> Mux5/2
  Interpreted MATLAB Function11/1 -> Mux5/1

== system Latest_Greatest_vSandberg/CMGs/CMG Steering Logic1/Subsystem ==
  "[A]" : Inport
  Divide : Product  Inputs=/*
  max (SVD[A]) : MATLABFcn  MATLABFcn=max(svd(u))
  min (SVD[A]) : MATLABFcn  MATLABFcn=min(svd(u))
  1/Cond[A] : Outport  VectorParamsAs1DForOutWhenUnconnected=off
  wires:
  Divide/1 -> 1/Cond[A]/1
  max (SVD[A])/1 -> Divide/2
  min (SVD[A])/1 -> Divide/1
  "[A]"/1 -> max (SVD[A])/1, min (SVD[A])/1

== system Latest_Greatest_vSandberg/CMGs/CMG Steering Logic1/Subsystem1 ==
  delta : Inport
  3x4 : Reshape  OutputDimensionality=Customize  OutputDimensions=[3,4]
  "[A] Matrix" : MATLABFcn  MATLABFcn="[ -cos(beta(1))*cos(u(1)),  sin(u(2)), cos(beta(3))*cos(u(3)), 0   ;  -sin(u(1)),  -cos(beta(2))*cos(u(2)),  sin(u(3)),   0;  sin(beta(1))*cos(u(1)),  sin(beta(2))*cos(u(2)),  sin(beta(3))*cos(u(3)),   0  ]"
  "[A]" : Outport  VectorParamsAs1DForOutWhenUnconnected=off
  wires:
  "[A] Matrix"/1 -> 3x4/1
  delta/1 -> "[A] Matrix"/1
  3x4/1 -> "[A]"/1

== system Latest_Greatest_vSandberg/CMGs/CMG Steering Logic1/Subsystem3 ==
  1/Cond[A] : Inport
  deltaDot : Inport  Port=2
  Switch : Switch  Threshold=2.21  SaturateOnIntegerOverflow=off  InputSameDT=off
  Unit Delay : UnitDelay  SampleTime=-1  HasFrameUpgradeWarning=on
  Out1 : Outport  VectorParamsAs1DForOutWhenUnconnected=off
  wires:
  1/Cond[A]/1 -> Switch/2
  deltaDot/1 -> Switch/1
  Switch/1 -> Unit Delay/1, Out1/1
  Unit Delay/1 -> Switch/3

== system Latest_Greatest_vSandberg/CMGs/Subsystem1/Displays ==
  Tc : Inport
  d : Inport  Port=2
  u : Inport  Port=3
  -3 : Gain  Gain=-1  SaturateOnIntegerOverflow=on  OutDataTypeStr=Inherit: Same as input  ParamDataTypeStr=Inherit: Same as input
  Demux : Demux
  Demux1 : Demux  Outputs=3
  Demux2 : Demux  Outputs=3
  Sum : Sum  Inputs=+-|
  Tcmg : Scope  NumInputPorts=3
  To Workspace : ToWorkspace  VariableName=ControlError  SampleTime=-1
  d. : Scope  NumInputPorts=4
  uc : Scope  NumInputPorts=3
  wires:
  d/1 -> Demux/1
  u/1 -> -3/1
  Demux/4 -> d./4
  Demux/3 -> d./3
  Demux/2 -> d./2
  Demux/1 -> d./1
  -3/1 -> Demux1/1, Sum/1
  Tc/1 -> Demux2/1, Sum/2
  Demux2/1 -> Tcmg/1
  Demux2/2 -> Tcmg/2
  Demux2/3 -> Tcmg/3
  Demux1/1 -> uc/1
  Demux1/2 -> uc/2
  Demux1/3 -> uc/3
  Sum/1 -> To Workspace/1

== system Latest_Greatest_vSandberg/CMGs/Subsystem1/Subsystem ==
  SAC/MP : Inport
  Demux : Demux  Outputs=8
  Mux : Mux  Inputs=3
  Mux1 : Mux
  To Workspace : ToWorkspace  VariableName=flag  SampleTime=-1
  Torque : Outport  VectorParamsAs1DForOutWhenUnconnected=off
  GimbalAngles : Outport  Port=2  VectorParamsAs1DForOutWhenUnconnected=off
  wires:
  SAC/MP/1 -> Demux/1
  Demux/8 -> To Workspace/1
  Demux/1 -> Mux/1
  Demux/2 -> Mux/2
  Demux/3 -> Mux/3
  Demux/4 -> Mux1/1
  Demux/5 -> Mux1/2
  Demux/6 -> Mux1/3
  Demux/7 -> Mux1/4
  Mux1/1 -> GimbalAngles/1
  Mux/1 -> Torque/1

== system Latest_Greatest_vSandberg/CMGs/Subsystem1/Subsystem2 ==
  note: Gimbal Angles
  note: u
  note: flag
  u : Inport
  gimbal angles : Inport  Port=2
  Constant1 : Constant
  Mux1 : Mux  Inputs=3
  MP : Outport  VectorParamsAs1DForOutWhenUnconnected=off
  wires:
  u/1 -> Mux1/1
  Constant1/1 -> Mux1/3
  Mux1/1 -> MP/1
  gimbal angles/1 -> Mux1/2

== system Latest_Greatest_vSandberg/CMGs/Subsystem3/Subsystem1 ==
  note: Note if you actually go into these blocks, theyre actually -Ki etc
  note: e(s)
  note: w
  note: (s)
  note: q
  note: (s)
  note: u(s)
  note: *
  note: q
  note: (s)
  note: w
  note: *
  note: (s)
  Full State Feedback : Inport
  FullCMDTraj : Inport  Port=2
  Demux : Demux  Outputs=2
  Demux1 : Demux  Outputs=2
  Gain : Gain  Gain=Ki
  Gain1 : Gain  Gain=Kp
  Gain2 : Gain  Gain=Kd
  Gain3 : Gain  Multiplication=Matrix(K*u)
  Integrator9 : Integrator
  Subsystem25 : Subsystem  Commented=on
      mask Display: disp('Ki')
  Subsystem26 : Subsystem  Commented=on
      mask Display: disp('Kp')
  Subsystem27 : Subsystem  Commented=on
      mask Display: disp('Kd')
  Sum12 : Sum  Inputs=|+-
  Sum14 : Sum  Inputs=+++
  Sum15 : Sum  Inputs=|+-
  "Control, u-fb" : Outport  VectorParamsAs1DForOutWhenUnconnected=off
  wires:
  Demux/1 -> Sum12/2
  Sum15/1 -> Gain2/1
  Integrator9/1 -> Gain/1
  Sum12/1 -> Gain1/1, Integrator9/1
  Gain2/1 -> Sum14/3
  Gain1/1 -> Sum14/2
  Gain/1 -> Sum14/1
  Demux1/2 -> Sum15/1
  Demux1/1 -> Sum12/1
  Full State Feedback/1 -> Demux/1
  Demux/2 -> Sum15/2
  FullCMDTraj/1 -> Demux1/1
  Sum14/1 -> Gain3/1
  Gain3/1 -> "Control, u-fb"/1

== system Latest_Greatest_vSandberg/CMGs/Subsystem3/Subsystem2 ==
  note: DOUBLE CHECK WHICH SIGN THIS SUM SHOULD BE, BELIEVE IT IS NOW CORRECT
  note: (s)
  note: *
  note: w
  note: (s)
  note: q
  note: *
  note: u(s)
  note: (s)
  note: q
  note: (s)
  note: w
  note: e(s)
  note: Note if you actually go into these blocks, theyre actually -Ki etc
  Full State Feedback : Inport
  FullCMDTraj : Inport  Port=2
  Cross Product : vrlib/Utilities/Cross Product
  Demux : Demux  Outputs=2
  Demux1 : Demux  Outputs=2
  Gain : Gain  Gain=Ki
  Gain1 : Gain  Gain=Kp
  Gain2 : Gain  Gain=Kd
  Gain3 : Gain  Gain=Kd
  Gain4 : Gain  Gain=Imo  Multiplication=Matrix(K*u)
  Integrator9 : Integrator
  Scope : Scope
  Scope1 : Scope
  Sum : Sum  Inputs=|++
  Sum12 : Sum  Inputs=|+-
  Sum14 : Sum  Inputs=+++
  Sum15 : Sum  Inputs=|+-
  "Control, u-fb" : Outport  VectorParamsAs1DForOutWhenUnconnected=off
  wires:
  Sum/1 -> "Control, u-fb"/1
  Sum14/1 -> Sum/1
  FullCMDTraj/1 -> Demux1/1
  Demux/2 -> Sum15/2
  Full State Feedback/1 -> Demux/1
  Demux1/1 -> Sum12/1
  Gain/1 -> Sum14/1
  Gain1/1 -> Sum14/2
  Gain2/1 -> Sum14/3
  Sum12/1 -> Integrator9/1, Gain1/1
  Integrator9/1 -> Gain/1
  Sum15/1 -> Gain2/1
  Demux/1 -> Sum12/2
  Gain4/1 -> Cross Product/2
  Cross Product/1 -> Gain3/1
  Gain3/1 -> Scope/1, Sum/2
  Demux1/2 -> Gain4/1, Cross Product/1, Sum15/1, Scope1/1

== system Latest_Greatest_vSandberg/CMGs/Subsystem3/Subsystem4 ==
  note: The derivative block even though not being used, could e throwing numerical errors
  note: Interestingly, my version+ PDI is better than Toolman's in phi, 0.1 vs 0.05 error. However the errors in the other two axes are just slightly higher DURING the maneuver, however how are the final values?
  note: $\dot q_d$
  note: $q_d$
  note: Find paper where the reference trajectory is not used, must have taken the derivative of qdot
  note: Accounts and adapts for error in Inertia Matrix
  note: Does not account for Errors in Inertia Matrix
  note: *
  note: (s)
  note: w
  LAMBDA*xtilda : Inport
  w : Inport  Port=2
  State Feedback : Inport  Port=3
  Trajectory Desired : Inport  Port=4
  Demux : Demux  Outputs=2
  Demux1 : Demux  Outputs=2
  Manual Switch : ManualSwitch
  Manual Switch1 : ManualSwitch
  Manual Switch2 : ManualSwitch  CurrentSetting=0
  Scope : Scope
  Subsystem : Subsystem
      mask Display: disp('Classical Feedforward')
  Subsystem1 : Subsystem
      mask Display: disp('Adaptive Feedforward')
  Subsystem2 : Subsystem
      mask Display: disp('Adaptive Feedforward \n Sandberg')
  Subsystem3 : Subsystem
      mask Display: disp('DAI')
  Sum : Sum  Inputs=|+-
  uFF : Outport  VectorParamsAs1DForOutWhenUnconnected=off
  wires:
  w/1 -> Subsystem1/2(w), Subsystem/2(In2)
  [OmegaDotTrajectory] -> Subsystem1/1(omegadot_traj), Subsystem/1(In1)
  Subsystem/1(Out1) -> Sum/1, Manual Switch/1
  LAMBDA*xtilda/1 -> Subsystem1/3(LAMBDA*xtilda)
  Subsystem1/1(Out1) -> Manual Switch/2
  Demux1/1 -> Subsystem3/1(q), Subsystem2/1(q)
  Demux1/2 -> Subsystem3/2(qdot), Subsystem2/2(qdot)
  Demux/1 -> Subsystem3/3(q_d), Subsystem2/3(q_d)
  [OmegaDotTrajectory] -> Subsystem2/5(qdotdot_d), Subsystem3/5(qdotdot_d)
  Manual Switch/1 -> Manual Switch1/1
  Demux/2 -> Subsystem3/4(qdot_d), Subsystem2/4(qdot_d)
  Trajectory Desired/1 -> Demux/1
  State Feedback/1 -> Demux1/1
  Subsystem2/1(uFF1) -> Sum/2, Manual Switch1/2
  Manual Switch1/1 -> Manual Switch2/1
  Subsystem3/1(uFF1) -> Manual Switch2/2
  Manual Switch2/1 -> uFF/1
  Sum/1 -> Scope/1

== system Latest_Greatest_vSandberg/Subsystem2/Subsystem/Gravity Gradient ==
  note: Gravity Gradient Disturbances
  DCM : Inport
  3*mu/Ro^3 : Gain  Gain=3*mu/(h+Re)^3  Multiplication=Matrix(K*u)  SaturateOnIntegerOverflow=on  OutDataTypeStr=Inherit: Same as input  ParamDataTypeStr=Inherit: Same as input
  3x3 cross product : aerospace/Axes Transformations/3x3 cross product
  Body Inertia : Gain  Gain=Imo  Multiplication=Matrix(K*u)  SaturateOnIntegerOverflow=on  OutDataTypeStr=Inherit: Same as input  ParamDataTypeStr=Inherit: Same as input
  Select ci3 : Subsystem
  Tgg : Outport
  wires:
  DCM/1 -> Select ci3/1(U)
  Select ci3/1(U(E)) -> Body Inertia/1, 3x3 cross product/1
  3x3 cross product/1 -> 3*mu/Ro^3/1
  3*mu/Ro^3/1 -> Tgg/1
  Body Inertia/1 -> 3x3 cross product/2

== system Latest_Greatest_vSandberg/Subsystem2/Subsystem/Magnetic Torque ==
  note: Bxo
  note: Byo
  note: Bzo
  note: Magnetic Disturbances
  DCM : Inport
  alpha : Inport  Port=2
  inclination : Inport  Port=3
  u : Inport  Port=4
  . : aerospace/Axes Transformations/3x3 cross product
  .K/R^3 : Gain  Gain=K/R^3  SaturateOnIntegerOverflow=on  OutDataTypeStr=Inherit: Same as input  ParamDataTypeStr=Inherit: Same as input
  Cx (orbit coordinates) : Fcn  Expr="cos(u[2])* ( cos(u[4])*sin(u[3])-sin(u[4])*cos(u[3])*cos(u[1])  ) - sin(u[2])*sin(u[4])*sin(u[1])"
  Cx (body coordinates) : Fcn  Expr=u[1]*u[10]+u[2]*u[11]+u[3]*u[12]
  Cy (orbit coordinates) : Fcn  Expr=-cos(u[4])*cos(u[3])-sin(u[4])*sin(u[3])*cos(u[1])
  Cy (body coordinates) : Fcn  Expr=u[4]*u[10]+u[5]*u[11]+u[6]*u[12]
  Cz (orbit coordinates) : Fcn  Expr="2*sin(u[2])*  (cos(u[4])*sin(u[3])-sin(u[4])*cos(u[3])*cos(u[1]) ) + 2*cos(u[2])*sin(u[4])*sin(u[1])"
  Cz (body coordinates) : Fcn  Expr=u[7]*u[10]+u[8]*u[11]+u[9]*u[12]
  K/R^3 : Gain  Gain=K/R^3  SaturateOnIntegerOverflow=on  OutDataTypeStr=Inherit: Same as input  ParamDataTypeStr=Inherit: Same as input
  K/R^3. : Gain  Gain=K/R^3  SaturateOnIntegerOverflow=on  OutDataTypeStr=Inherit: Same as input  ParamDataTypeStr=Inherit: Same as input
  Magnetic B Field : Scope  NumInputPorts=3
  Magnetic B Field in Body Coords : Scope
  Magnetic Residual : Constant  Value=M
  Mux : Mux
  Mux1 : Mux
  Mux2 : Mux  Inputs=3
  epsilon : Constant  Value=epsilon
  Sb : Outport
  wires:
  u/1 -> Mux/1
  alpha/1 -> Mux/2
  inclination/1 -> Mux/3
  Mux/1 -> Cy (orbit coordinates)/1, Cx (orbit coordinates)/1, Cz (orbit coordinates)/1
  epsilon/1 -> Mux/4
  Cx (orbit coordinates)/1 -> K/R^3/1
  Cy (orbit coordinates)/1 -> K/R^3./1
  Cz (orbit coordinates)/1 -> .K/R^3/1
  DCM/1 -> Mux1/1
  K/R^3/1 -> Mux1/2, Magnetic B Field/1
  K/R^3./1 -> Mux1/3, Magnetic B Field/2
  .K/R^3/1 -> Mux1/4, Magnetic B Field/3
  Mux1/1 -> Cy (body coordinates)/1, Cx (body coordinates)/1, Cz (body coordinates)/1
  Cy (body coordinates)/1 -> Mux2/2
  Cx (body coordinates)/1 -> Mux2/1
  Cz (body coordinates)/1 -> Mux2/3
  ./1 -> Sb/1
  Magnetic Residual/1 -> ./1
  Mux2/1 -> ./2, Magnetic B Field in Body Coords/1

== system Latest_Greatest_vSandberg/Subsystem2/Subsystem/Orbit parameters ==
  note: alpha
  note: nu=nuo-alpha
  note: Orbit parameters
  Clock : Clock
  Sum2 : Sum  Inputs=-+  InputSameDT=on  SaturateOnIntegerOverflow=on  OutDataTypeStr=Inherit: Same as first input
  Sum3 : Sum  InputSameDT=on  SaturateOnIntegerOverflow=on  OutDataTypeStr=Inherit: Same as first input
  Sum4 : Sum  InputSameDT=on  SaturateOnIntegerOverflow=on  OutDataTypeStr=Inherit: Same as first input
  alphao : Constant  Value=alphao
  inclination : Constant  Value=incln
  nuo : Constant  Value=nuo
  udot*t=t/365/360 : Gain  Gain=1/365.242/360  SaturateOnIntegerOverflow=on  OutDataTypeStr=Inherit: Same as input  ParamDataTypeStr=Inherit: Same as input
  uo : Constant  Value=uo
  wo : Gain  Gain=wo  SaturateOnIntegerOverflow=on  OutDataTypeStr=Inherit: Same as input  ParamDataTypeStr=Inherit: Same as input
  alpha : Outport
  incln : Outport  Port=2
  u : Outport  Port=3
  nu : Outport  Port=4
  wires:
  Clock/1 -> wo/1, udot*t=t/365/360/1
  alphao/1 -> Sum4/1
  wo/1 -> Sum4/2
  udot*t=t/365/360/1 -> Sum3/1
  uo/1 -> Sum3/2
  nuo/1 -> Sum2/1
  Sum4/1 -> Sum2/2, alpha/1
  Sum2/1 -> nu/1
  inclination/1 -> incln/1
  Sum3/1 -> u/1
